simulink model "TST_ExtDem_SetPoint"  (R2016b)
settings: Solver=FixedStepDiscrete  StartTime=0.0  StopTime=simTime  FixedStep=sampleTime  RelTol=1e-3
values from neighbouring files (symbols this model uses):
  testCase = 1    [initTST_ExtDem_SetPoint_001.m]    (also in initTST_ExtDem_SetPoint_002.m = 2; initTST_ExtDem_SetPoint_003.m = 3)
libraries: simulink x13, UnitTest_Lib x9
settings Model: Creator=bianxuyin  LastModifiedBy=bianxuyin
settings DebuggingCC: SignalRangeChecking=error

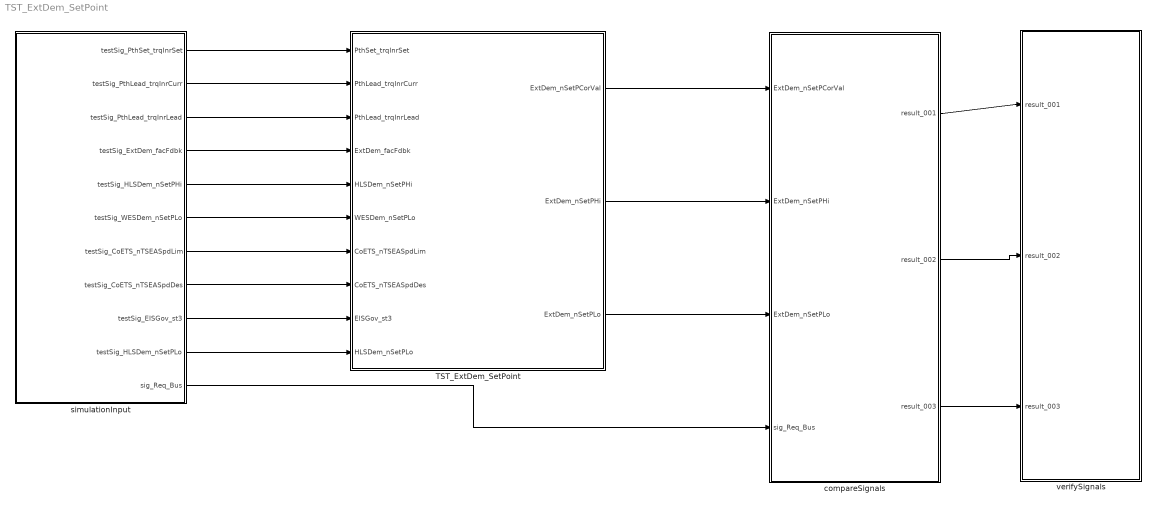
== system TST_ExtDem_SetPoint ==
  TST_ExtDem_SetPoint : Subsystem
  compareSignals : Subsystem
  simulationInput : Subsystem
  verifySignals : Subsystem
  wires:
  simulationInput/1(testSig_PthSet_trqInrSet) -> TST_ExtDem_SetPoint/1(PthSet_trqInrSet)
  simulationInput/2(testSig_PthLead_trqInrCurr) -> TST_ExtDem_SetPoint/2(PthLead_trqInrCurr)
  simulationInput/3(testSig_PthLead_trqInrLead) -> TST_ExtDem_SetPoint/3(PthLead_trqInrLead)
  simulationInput/4(testSig_ExtDem_facFdbk) -> TST_ExtDem_SetPoint/4(ExtDem_facFdbk)
  simulationInput/5(testSig_HLSDem_nSetPHi) -> TST_ExtDem_SetPoint/5(HLSDem_nSetPHi)
  simulationInput/6(testSig_WESDem_nSetPLo) -> TST_ExtDem_SetPoint/6(WESDem_nSetPLo)
  simulationInput/7(testSig_CoETS_nTSEASpdLim) -> TST_ExtDem_SetPoint/7(CoETS_nTSEASpdLim)
  simulationInput/8(testSig_CoETS_nTSEASpdDes) -> TST_ExtDem_SetPoint/8(CoETS_nTSEASpdDes)
  simulationInput/9(testSig_EISGov_st3) -> TST_ExtDem_SetPoint/9(EISGov_st3)
  simulationInput/10(testSig_HLSDem_nSetPLo) -> TST_ExtDem_SetPoint/10(HLSDem_nSetPLo)
  TST_ExtDem_SetPoint/1(ExtDem_nSetPCorVal) -> compareSignals/1(ExtDem_nSetPCorVal)
  TST_ExtDem_SetPoint/2(ExtDem_nSetPHi) -> compareSignals/2(ExtDem_nSetPHi)
  TST_ExtDem_SetPoint/3(ExtDem_nSetPLo) -> compareSignals/3(ExtDem_nSetPLo)
  simulationInput/11(sig_Req_Bus) -> compareSignals/4(sig_Req_Bus)
  compareSignals/1(result_001) -> verifySignals/1(result_001)
  compareSignals/2(result_002) -> verifySignals/2(result_002)
  compareSignals/3(result_003) -> verifySignals/3(result_003)

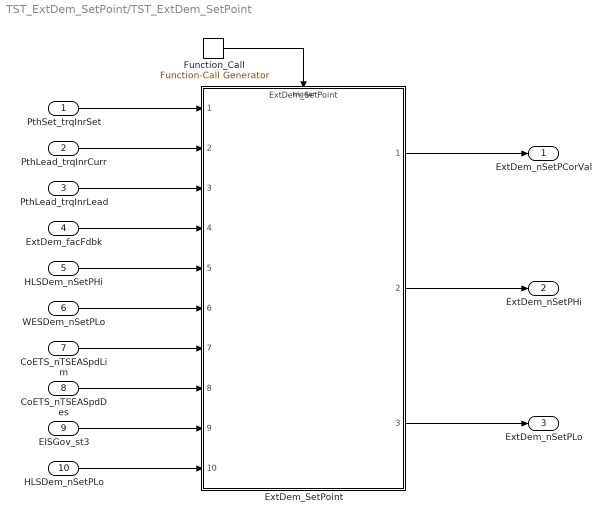
== system TST_ExtDem_SetPoint/TST_ExtDem_SetPoint ==
  PthSet_trqInrSet : Inport
  PthLead_trqInrCurr : Inport  Port=2
  PthLead_trqInrLead : Inport  Port=3
  ExtDem_facFdbk : Inport  Port=4
  HLSDem_nSetPHi : Inport  Port=5
  WESDem_nSetPLo : Inport  Port=6
  CoETS_nTSEASpdLim : Inport  Port=7
  CoETS_nTSEASpdDes : Inport  Port=8
  EISGov_st3 : Inport  Port=9
  HLSDem_nSetPLo : Inport  Port=10
  ExtDem_SetPoint : ModelReference  ModelNameDialog=ExtDem_SetPoint  SimulationMode=Normal  ModelReferenceVersion=1.39  TriggerPortName=function  TriggerPortTriggerType=function-call  TriggerPortStatesWhenEnabling=held
  Function_Call : simulink/Ports & Subsystems/Function-Call Generator  sample_time=sampleTime  numberOfIterations=1
  ExtDem_nSetPCorVal : Outport
  ExtDem_nSetPHi : Outport  Port=2
  ExtDem_nSetPLo : Outport  Port=3
  wires:
  Function_Call/1 -> ExtDem_SetPoint/Trigger
  PthSet_trqInrSet/1 -> ExtDem_SetPoint/1
  PthLead_trqInrCurr/1 -> ExtDem_SetPoint/2
  PthLead_trqInrLead/1 -> ExtDem_SetPoint/3
  ExtDem_facFdbk/1 -> ExtDem_SetPoint/4
  HLSDem_nSetPHi/1 -> ExtDem_SetPoint/5
  WESDem_nSetPLo/1 -> ExtDem_SetPoint/6
  CoETS_nTSEASpdLim/1 -> ExtDem_SetPoint/7
  CoETS_nTSEASpdDes/1 -> ExtDem_SetPoint/8
  EISGov_st3/1 -> ExtDem_SetPoint/9
  HLSDem_nSetPLo/1 -> ExtDem_SetPoint/10
  ExtDem_SetPoint/1 -> ExtDem_nSetPCorVal/1
  ExtDem_SetPoint/2 -> ExtDem_nSetPHi/1
  ExtDem_SetPoint/3 -> ExtDem_nSetPLo/1

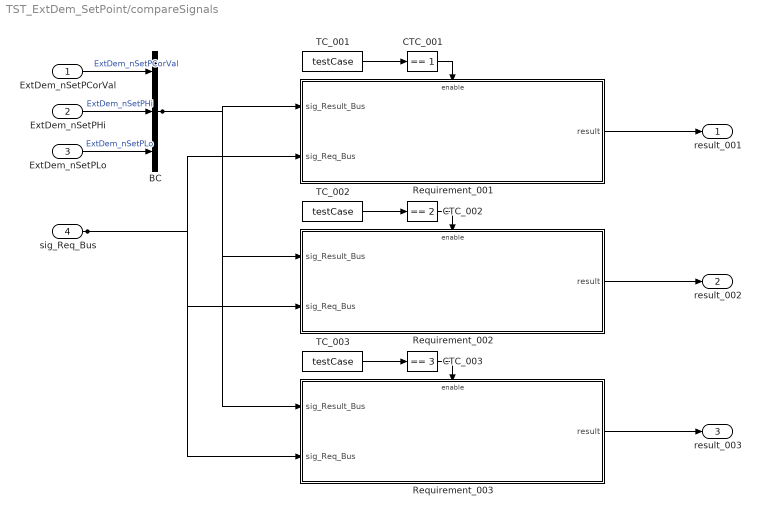
== system TST_ExtDem_SetPoint/compareSignals ==
  ExtDem_nSetPCorVal : Inport
  ExtDem_nSetPHi : Inport  Port=2
  ExtDem_nSetPLo : Inport  Port=3
  sig_Req_Bus : Inport  Port=4
  BC : BusCreator  Inputs=3
  CTC_001 : simulink/Logic and Bit Operations/Compare To Constant  relop===  const=1  OutDataTypeStr=boolean
  CTC_002 : simulink/Logic and Bit Operations/Compare To Constant  relop===  const=2  OutDataTypeStr=boolean
  CTC_003 : simulink/Logic and Bit Operations/Compare To Constant  relop===  const=3  OutDataTypeStr=boolean
  Requirement_001 : Subsystem
  Requirement_002 : Subsystem
  Requirement_003 : Subsystem
  TC_001 : Constant  Value=testCase
  TC_002 : Constant  Value=testCase
  TC_003 : Constant  Value=testCase
  result_001 : Outport
  result_002 : Outport  Port=2
  result_003 : Outport  Port=3
  wires:
  ExtDem_nSetPCorVal/1 -> BC/1  "ExtDem_nSetPCorVal"
  ExtDem_nSetPHi/1 -> BC/2  "ExtDem_nSetPHi"
  ExtDem_nSetPLo/1 -> BC/3  "ExtDem_nSetPLo"
  TC_001/1 -> CTC_001/1
  CTC_001/1 -> Requirement_001/Enable
  sig_Req_Bus/1 -> Requirement_001/2(sig_Req_Bus), Requirement_002/2(sig_Req_Bus), Requirement_003/2(sig_Req_Bus)
  BC/1 -> Requirement_001/1(sig_Result_Bus), Requirement_002/1(sig_Result_Bus), Requirement_003/1(sig_Result_Bus)
  Requirement_001/1(result) -> result_001/1
  TC_002/1 -> CTC_002/1
  CTC_002/1 -> Requirement_002/Enable
  Requirement_002/1(result) -> result_002/1
  TC_003/1 -> CTC_003/1
  CTC_003/1 -> Requirement_003/Enable
  Requirement_003/1(result) -> result_003/1

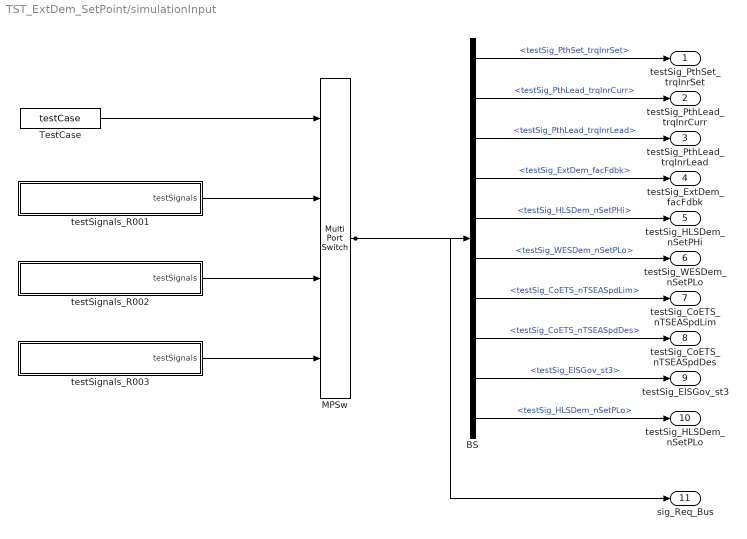
== system TST_ExtDem_SetPoint/simulationInput ==
  BS : BusSelector  OutputSignals=testSig_PthSet_trqInrSet,testSig_PthLead_trqInrCurr,testSig_PthLead_trqInrLead,testSig_ExtDem_facFdbk,testSig_HLSDem_nSetPHi,testSig_WESDem_nSetPLo,testSig_CoETS_nTSEASpdLim,testSig_CoETS_nTSEASpdDes,testSig_EISGov_st3,testSig_HLSDem_nSetPLo
  MPSw : MultiPortSwitch  SaturateOnIntegerOverflow=on  InputSameDT=on
  TestCase : Constant  Value=testCase
  testSignals_R001 : Subsystem
  testSignals_R002 : Subsystem
  testSignals_R003 : Subsystem
  testSig_PthSet_trqInrSet : Outport
  testSig_PthLead_trqInrCurr : Outport  Port=2
  testSig_PthLead_trqInrLead : Outport  Port=3
  testSig_ExtDem_facFdbk : Outport  Port=4
  testSig_HLSDem_nSetPHi : Outport  Port=5
  testSig_WESDem_nSetPLo : Outport  Port=6
  testSig_CoETS_nTSEASpdLim : Outport  Port=7
  testSig_CoETS_nTSEASpdDes : Outport  Port=8
  testSig_EISGov_st3 : Outport  Port=9
  testSig_HLSDem_nSetPLo : Outport  Port=10
  sig_Req_Bus : Outport  Port=11
  wires:
  BS/1 -> testSig_PthSet_trqInrSet/1  "<testSig_PthSet_trqInrSet>"
  BS/2 -> testSig_PthLead_trqInrCurr/1  "<testSig_PthLead_trqInrCurr>"
  BS/3 -> testSig_PthLead_trqInrLead/1  "<testSig_PthLead_trqInrLead>"
  BS/4 -> testSig_ExtDem_facFdbk/1  "<testSig_ExtDem_facFdbk>"
  BS/5 -> testSig_HLSDem_nSetPHi/1  "<testSig_HLSDem_nSetPHi>"
  BS/6 -> testSig_WESDem_nSetPLo/1  "<testSig_WESDem_nSetPLo>"
  BS/7 -> testSig_CoETS_nTSEASpdLim/1  "<testSig_CoETS_nTSEASpdLim>"
  BS/8 -> testSig_CoETS_nTSEASpdDes/1  "<testSig_CoETS_nTSEASpdDes>"
  BS/9 -> testSig_EISGov_st3/1  "<testSig_EISGov_st3>"
  BS/10 -> testSig_HLSDem_nSetPLo/1  "<testSig_HLSDem_nSetPLo>"
  MPSw/1 -> BS/1, sig_Req_Bus/1
  TestCase/1 -> MPSw/1
  testSignals_R001/1(testSignals) -> MPSw/2
  testSignals_R002/1(testSignals) -> MPSw/3
  testSignals_R003/1(testSignals) -> MPSw/4

== system TST_ExtDem_SetPoint/verifySignals ==
  result_001 : Inport
  result_002 : Inport  Port=2
  result_003 : Inport  Port=3
  Assertion_001 : Assertion  Enabled=off
  Assertion_002 : Assertion  Enabled=off
  Assertion_003 : Assertion  Enabled=off
  wires:
  result_001/1 -> Assertion_001/1
  result_002/1 -> Assertion_002/1
  result_003/1 -> Assertion_003/1

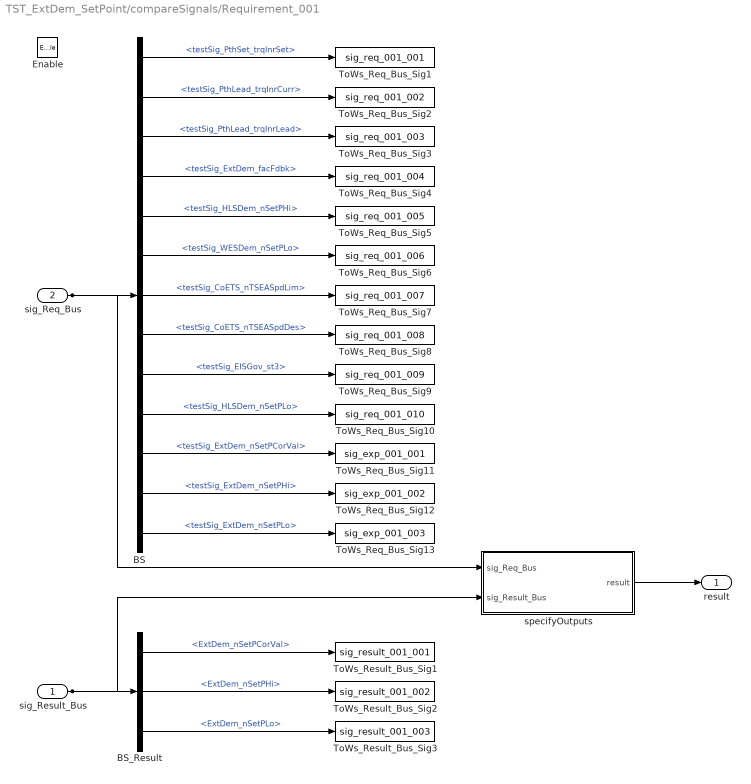
== system TST_ExtDem_SetPoint/compareSignals/Requirement_001 ==
  sig_Result_Bus : Inport
  sig_Req_Bus : Inport  Port=2
  Enable : EnablePort
  BS : BusSelector  OutputSignals=testSig_PthSet_trqInrSet,testSig_PthLead_trqInrCurr,testSig_PthLead_trqInrLead,testSig_ExtDem_facFdbk,testSig_HLSDem_nSetPHi,testSig_WESDem_nSetPLo,testSig_CoETS_nTSEASpdLim,testSig_CoETS_nTSEASpdDes,testSig_EISGov_st3,testSig_HLSDem_nSetPLo,testSig_ExtDem_nSetPCorVal,testSig_ExtDem_nSetPHi,testSig_ExtDem_nSetPLo
  BS_Result : BusSelector  OutputSignals=ExtDem_nSetPCorVal,ExtDem_nSetPHi,ExtDem_nSetPLo
  ToWs_Req_Bus_Sig1 : ToWorkspace  VariableName=sig_req_001_001  SaveFormat=Structure With Time
  ToWs_Req_Bus_Sig10 : ToWorkspace  VariableName=sig_req_001_010  SaveFormat=Structure With Time
  ToWs_Req_Bus_Sig11 : ToWorkspace  VariableName=sig_exp_001_001  SaveFormat=Structure With Time
  ToWs_Req_Bus_Sig12 : ToWorkspace  VariableName=sig_exp_001_002  SaveFormat=Structure With Time
  ToWs_Req_Bus_Sig13 : ToWorkspace  VariableName=sig_exp_001_003  SaveFormat=Structure With Time
  ToWs_Req_Bus_Sig2 : ToWorkspace  VariableName=sig_req_001_002  SaveFormat=Structure With Time
  ToWs_Req_Bus_Sig3 : ToWorkspace  VariableName=sig_req_001_003  SaveFormat=Structure With Time
  ToWs_Req_Bus_Sig4 : ToWorkspace  VariableName=sig_req_001_004  SaveFormat=Structure With Time
  ToWs_Req_Bus_Sig5 : ToWorkspace  VariableName=sig_req_001_005  SaveFormat=Structure With Time
  ToWs_Req_Bus_Sig6 : ToWorkspace  VariableName=sig_req_001_006  SaveFormat=Structure With Time
  ToWs_Req_Bus_Sig7 : ToWorkspace  VariableName=sig_req_001_007  SaveFormat=Structure With Time
  ToWs_Req_Bus_Sig8 : ToWorkspace  VariableName=sig_req_001_008  SaveFormat=Structure With Time
  ToWs_Req_Bus_Sig9 : ToWorkspace  VariableName=sig_req_001_009  SaveFormat=Structure With Time
  ToWs_Result_Bus_Sig1 : ToWorkspace  VariableName=sig_result_001_001  SaveFormat=Structure With Time
  ToWs_Result_Bus_Sig2 : ToWorkspace  VariableName=sig_result_001_002  SaveFormat=Structure With Time
  ToWs_Result_Bus_Sig3 : ToWorkspace  VariableName=sig_result_001_003  SaveFormat=Structure With Time
  specifyOutputs : Subsystem
  result : Outport
  wires:
  sig_Req_Bus/1 -> BS/1, specifyOutputs/1(sig_Req_Bus)
  BS/1 -> ToWs_Req_Bus_Sig1/1  "<testSig_PthSet_trqInrSet>"
  BS/2 -> ToWs_Req_Bus_Sig2/1  "<testSig_PthLead_trqInrCurr>"
  BS/3 -> ToWs_Req_Bus_Sig3/1  "<testSig_PthLead_trqInrLead>"
  BS/4 -> ToWs_Req_Bus_Sig4/1  "<testSig_ExtDem_facFdbk>"
  BS/5 -> ToWs_Req_Bus_Sig5/1  "<testSig_HLSDem_nSetPHi>"
  BS/6 -> ToWs_Req_Bus_Sig6/1  "<testSig_WESDem_nSetPLo>"
  BS/7 -> ToWs_Req_Bus_Sig7/1  "<testSig_CoETS_nTSEASpdLim>"
  BS/8 -> ToWs_Req_Bus_Sig8/1  "<testSig_CoETS_nTSEASpdDes>"
  BS/9 -> ToWs_Req_Bus_Sig9/1  "<testSig_EISGov_st3>"
  BS/10 -> ToWs_Req_Bus_Sig10/1  "<testSig_HLSDem_nSetPLo>"
  BS/11 -> ToWs_Req_Bus_Sig11/1  "<testSig_ExtDem_nSetPCorVal>"
  BS/12 -> ToWs_Req_Bus_Sig12/1  "<testSig_ExtDem_nSetPHi>"
  BS/13 -> ToWs_Req_Bus_Sig13/1  "<testSig_ExtDem_nSetPLo>"
  sig_Result_Bus/1 -> BS_Result/1, specifyOutputs/2(sig_Result_Bus)
  BS_Result/1 -> ToWs_Result_Bus_Sig1/1  "<ExtDem_nSetPCorVal>"
  BS_Result/2 -> ToWs_Result_Bus_Sig2/1  "<ExtDem_nSetPHi>"
  BS_Result/3 -> ToWs_Result_Bus_Sig3/1  "<ExtDem_nSetPLo>"
  specifyOutputs/1(result) -> result/1

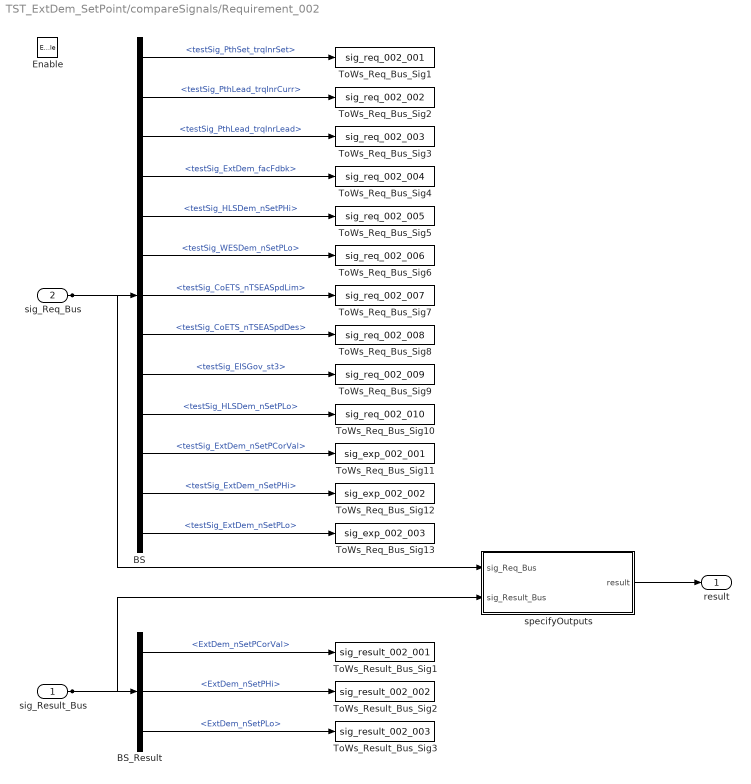
== system TST_ExtDem_SetPoint/compareSignals/Requirement_002 ==
  sig_Result_Bus : Inport
  sig_Req_Bus : Inport  Port=2
  Enable : EnablePort
  BS : BusSelector  OutputSignals=testSig_PthSet_trqInrSet,testSig_PthLead_trqInrCurr,testSig_PthLead_trqInrLead,testSig_ExtDem_facFdbk,testSig_HLSDem_nSetPHi,testSig_WESDem_nSetPLo,testSig_CoETS_nTSEASpdLim,testSig_CoETS_nTSEASpdDes,testSig_EISGov_st3,testSig_HLSDem_nSetPLo,testSig_ExtDem_nSetPCorVal,testSig_ExtDem_nSetPHi,testSig_ExtDem_nSetPLo
  BS_Result : BusSelector  OutputSignals=ExtDem_nSetPCorVal,ExtDem_nSetPHi,ExtDem_nSetPLo
  ToWs_Req_Bus_Sig1 : ToWorkspace  VariableName=sig_req_002_001  SaveFormat=Structure With Time
  ToWs_Req_Bus_Sig10 : ToWorkspace  VariableName=sig_req_002_010  SaveFormat=Structure With Time
  ToWs_Req_Bus_Sig11 : ToWorkspace  VariableName=sig_exp_002_001  SaveFormat=Structure With Time
  ToWs_Req_Bus_Sig12 : ToWorkspace  VariableName=sig_exp_002_002  SaveFormat=Structure With Time
  ToWs_Req_Bus_Sig13 : ToWorkspace  VariableName=sig_exp_002_003  SaveFormat=Structure With Time
  ToWs_Req_Bus_Sig2 : ToWorkspace  VariableName=sig_req_002_002  SaveFormat=Structure With Time
  ToWs_Req_Bus_Sig3 : ToWorkspace  VariableName=sig_req_002_003  SaveFormat=Structure With Time
  ToWs_Req_Bus_Sig4 : ToWorkspace  VariableName=sig_req_002_004  SaveFormat=Structure With Time
  ToWs_Req_Bus_Sig5 : ToWorkspace  VariableName=sig_req_002_005  SaveFormat=Structure With Time
  ToWs_Req_Bus_Sig6 : ToWorkspace  VariableName=sig_req_002_006  SaveFormat=Structure With Time
  ToWs_Req_Bus_Sig7 : ToWorkspace  VariableName=sig_req_002_007  SaveFormat=Structure With Time
  ToWs_Req_Bus_Sig8 : ToWorkspace  VariableName=sig_req_002_008  SaveFormat=Structure With Time
  ToWs_Req_Bus_Sig9 : ToWorkspace  VariableName=sig_req_002_009  SaveFormat=Structure With Time
  ToWs_Result_Bus_Sig1 : ToWorkspace  VariableName=sig_result_002_001  SaveFormat=Structure With Time
  ToWs_Result_Bus_Sig2 : ToWorkspace  VariableName=sig_result_002_002  SaveFormat=Structure With Time
  ToWs_Result_Bus_Sig3 : ToWorkspace  VariableName=sig_result_002_003  SaveFormat=Structure With Time
  specifyOutputs : Subsystem
  result : Outport
  wires:
  sig_Req_Bus/1 -> BS/1, specifyOutputs/1(sig_Req_Bus)
  BS/1 -> ToWs_Req_Bus_Sig1/1  "<testSig_PthSet_trqInrSet>"
  BS/2 -> ToWs_Req_Bus_Sig2/1  "<testSig_PthLead_trqInrCurr>"
  BS/3 -> ToWs_Req_Bus_Sig3/1  "<testSig_PthLead_trqInrLead>"
  BS/4 -> ToWs_Req_Bus_Sig4/1  "<testSig_ExtDem_facFdbk>"
  BS/5 -> ToWs_Req_Bus_Sig5/1  "<testSig_HLSDem_nSetPHi>"
  BS/6 -> ToWs_Req_Bus_Sig6/1  "<testSig_WESDem_nSetPLo>"
  BS/7 -> ToWs_Req_Bus_Sig7/1  "<testSig_CoETS_nTSEASpdLim>"
  BS/8 -> ToWs_Req_Bus_Sig8/1  "<testSig_CoETS_nTSEASpdDes>"
  BS/9 -> ToWs_Req_Bus_Sig9/1  "<testSig_EISGov_st3>"
  BS/10 -> ToWs_Req_Bus_Sig10/1  "<testSig_HLSDem_nSetPLo>"
  BS/11 -> ToWs_Req_Bus_Sig11/1  "<testSig_ExtDem_nSetPCorVal>"
  BS/12 -> ToWs_Req_Bus_Sig12/1  "<testSig_ExtDem_nSetPHi>"
  BS/13 -> ToWs_Req_Bus_Sig13/1  "<testSig_ExtDem_nSetPLo>"
  sig_Result_Bus/1 -> BS_Result/1, specifyOutputs/2(sig_Result_Bus)
  BS_Result/1 -> ToWs_Result_Bus_Sig1/1  "<ExtDem_nSetPCorVal>"
  BS_Result/2 -> ToWs_Result_Bus_Sig2/1  "<ExtDem_nSetPHi>"
  BS_Result/3 -> ToWs_Result_Bus_Sig3/1  "<ExtDem_nSetPLo>"
  specifyOutputs/1(result) -> result/1

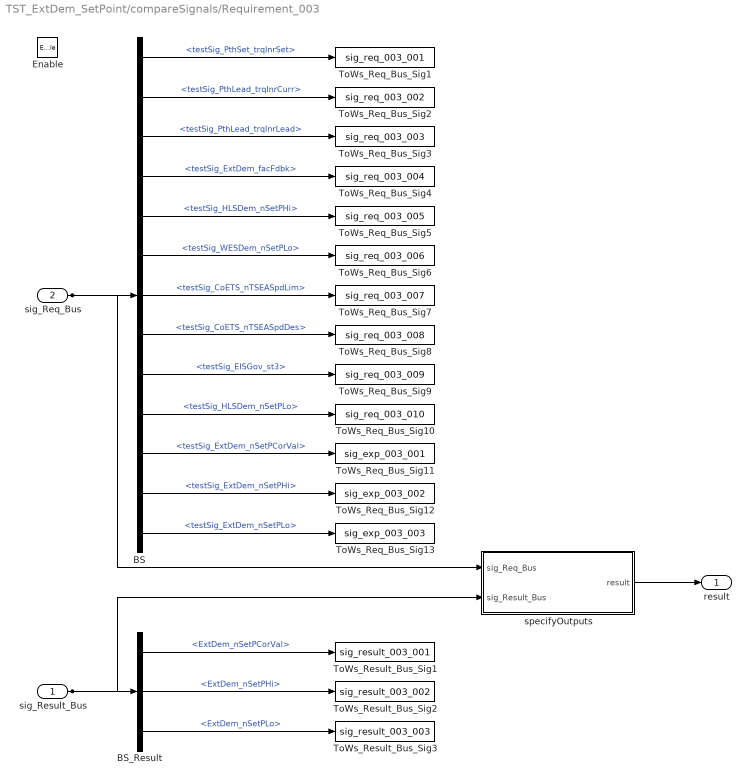
== system TST_ExtDem_SetPoint/compareSignals/Requirement_003 ==
  sig_Result_Bus : Inport
  sig_Req_Bus : Inport  Port=2
  Enable : EnablePort
  BS : BusSelector  OutputSignals=testSig_PthSet_trqInrSet,testSig_PthLead_trqInrCurr,testSig_PthLead_trqInrLead,testSig_ExtDem_facFdbk,testSig_HLSDem_nSetPHi,testSig_WESDem_nSetPLo,testSig_CoETS_nTSEASpdLim,testSig_CoETS_nTSEASpdDes,testSig_EISGov_st3,testSig_HLSDem_nSetPLo,testSig_ExtDem_nSetPCorVal,testSig_ExtDem_nSetPHi,testSig_ExtDem_nSetPLo
  BS_Result : BusSelector  OutputSignals=ExtDem_nSetPCorVal,ExtDem_nSetPHi,ExtDem_nSetPLo
  ToWs_Req_Bus_Sig1 : ToWorkspace  VariableName=sig_req_003_001  SaveFormat=Structure With Time
  ToWs_Req_Bus_Sig10 : ToWorkspace  VariableName=sig_req_003_010  SaveFormat=Structure With Time
  ToWs_Req_Bus_Sig11 : ToWorkspace  VariableName=sig_exp_003_001  SaveFormat=Structure With Time
  ToWs_Req_Bus_Sig12 : ToWorkspace  VariableName=sig_exp_003_002  SaveFormat=Structure With Time
  ToWs_Req_Bus_Sig13 : ToWorkspace  VariableName=sig_exp_003_003  SaveFormat=Structure With Time
  ToWs_Req_Bus_Sig2 : ToWorkspace  VariableName=sig_req_003_002  SaveFormat=Structure With Time
  ToWs_Req_Bus_Sig3 : ToWorkspace  VariableName=sig_req_003_003  SaveFormat=Structure With Time
  ToWs_Req_Bus_Sig4 : ToWorkspace  VariableName=sig_req_003_004  SaveFormat=Structure With Time
  ToWs_Req_Bus_Sig5 : ToWorkspace  VariableName=sig_req_003_005  SaveFormat=Structure With Time
  ToWs_Req_Bus_Sig6 : ToWorkspace  VariableName=sig_req_003_006  SaveFormat=Structure With Time
  ToWs_Req_Bus_Sig7 : ToWorkspace  VariableName=sig_req_003_007  SaveFormat=Structure With Time
  ToWs_Req_Bus_Sig8 : ToWorkspace  VariableName=sig_req_003_008  SaveFormat=Structure With Time
  ToWs_Req_Bus_Sig9 : ToWorkspace  VariableName=sig_req_003_009  SaveFormat=Structure With Time
  ToWs_Result_Bus_Sig1 : ToWorkspace  VariableName=sig_result_003_001  SaveFormat=Structure With Time
  ToWs_Result_Bus_Sig2 : ToWorkspace  VariableName=sig_result_003_002  SaveFormat=Structure With Time
  ToWs_Result_Bus_Sig3 : ToWorkspace  VariableName=sig_result_003_003  SaveFormat=Structure With Time
  specifyOutputs : Subsystem
  result : Outport
  wires:
  sig_Req_Bus/1 -> BS/1, specifyOutputs/1(sig_Req_Bus)
  BS/1 -> ToWs_Req_Bus_Sig1/1  "<testSig_PthSet_trqInrSet>"
  BS/2 -> ToWs_Req_Bus_Sig2/1  "<testSig_PthLead_trqInrCurr>"
  BS/3 -> ToWs_Req_Bus_Sig3/1  "<testSig_PthLead_trqInrLead>"
  BS/4 -> ToWs_Req_Bus_Sig4/1  "<testSig_ExtDem_facFdbk>"
  BS/5 -> ToWs_Req_Bus_Sig5/1  "<testSig_HLSDem_nSetPHi>"
  BS/6 -> ToWs_Req_Bus_Sig6/1  "<testSig_WESDem_nSetPLo>"
  BS/7 -> ToWs_Req_Bus_Sig7/1  "<testSig_CoETS_nTSEASpdLim>"
  BS/8 -> ToWs_Req_Bus_Sig8/1  "<testSig_CoETS_nTSEASpdDes>"
  BS/9 -> ToWs_Req_Bus_Sig9/1  "<testSig_EISGov_st3>"
  BS/10 -> ToWs_Req_Bus_Sig10/1  "<testSig_HLSDem_nSetPLo>"
  BS/11 -> ToWs_Req_Bus_Sig11/1  "<testSig_ExtDem_nSetPCorVal>"
  BS/12 -> ToWs_Req_Bus_Sig12/1  "<testSig_ExtDem_nSetPHi>"
  BS/13 -> ToWs_Req_Bus_Sig13/1  "<testSig_ExtDem_nSetPLo>"
  sig_Result_Bus/1 -> BS_Result/1, specifyOutputs/2(sig_Result_Bus)
  BS_Result/1 -> ToWs_Result_Bus_Sig1/1  "<ExtDem_nSetPCorVal>"
  BS_Result/2 -> ToWs_Result_Bus_Sig2/1  "<ExtDem_nSetPHi>"
  BS_Result/3 -> ToWs_Result_Bus_Sig3/1  "<ExtDem_nSetPLo>"
  specifyOutputs/1(result) -> result/1

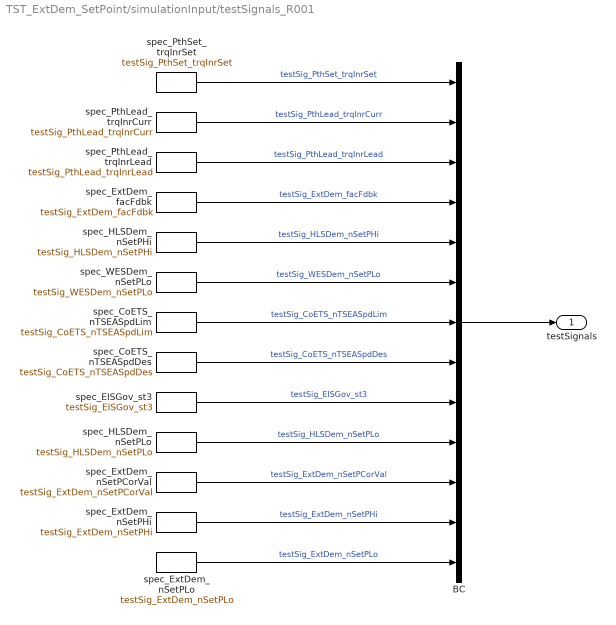
== system TST_ExtDem_SetPoint/simulationInput/testSignals_R001 ==
  BC : BusCreator  Inputs=13
  spec_CoETS_nTSEASpdDes : FromWorkspace  VariableName=testSig_CoETS_nTSEASpdDes  Interpolate=off  OutputAfterFinalValue=Holding final value
  spec_CoETS_nTSEASpdLim : FromWorkspace  VariableName=testSig_CoETS_nTSEASpdLim  Interpolate=off  OutputAfterFinalValue=Holding final value
  spec_EISGov_st3 : FromWorkspace  VariableName=testSig_EISGov_st3  Interpolate=off  OutputAfterFinalValue=Holding final value
  spec_ExtDem_facFdbk : FromWorkspace  VariableName=testSig_ExtDem_facFdbk  Interpolate=off  OutputAfterFinalValue=Holding final value
  spec_ExtDem_nSetPCorVal : FromWorkspace  VariableName=testSig_ExtDem_nSetPCorVal  Interpolate=off  OutputAfterFinalValue=Holding final value
  spec_ExtDem_nSetPHi : FromWorkspace  VariableName=testSig_ExtDem_nSetPHi  Interpolate=off  OutputAfterFinalValue=Holding final value
  spec_ExtDem_nSetPLo : FromWorkspace  VariableName=testSig_ExtDem_nSetPLo  Interpolate=off  OutputAfterFinalValue=Holding final value
  spec_HLSDem_nSetPHi : FromWorkspace  VariableName=testSig_HLSDem_nSetPHi  Interpolate=off  OutputAfterFinalValue=Holding final value
  spec_HLSDem_nSetPLo : FromWorkspace  VariableName=testSig_HLSDem_nSetPLo  Interpolate=off  OutputAfterFinalValue=Holding final value
  spec_PthLead_trqInrCurr : FromWorkspace  VariableName=testSig_PthLead_trqInrCurr  Interpolate=off  OutputAfterFinalValue=Holding final value
  spec_PthLead_trqInrLead : FromWorkspace  VariableName=testSig_PthLead_trqInrLead  Interpolate=off  OutputAfterFinalValue=Holding final value
  spec_PthSet_trqInrSet : FromWorkspace  VariableName=testSig_PthSet_trqInrSet  Interpolate=off  OutputAfterFinalValue=Holding final value
  spec_WESDem_nSetPLo : FromWorkspace  VariableName=testSig_WESDem_nSetPLo  Interpolate=off  OutputAfterFinalValue=Holding final value
  testSignals : Outport
  wires:
  BC/1 -> testSignals/1
  spec_PthSet_trqInrSet/1 -> BC/1  "testSig_PthSet_trqInrSet"
  spec_PthLead_trqInrCurr/1 -> BC/2  "testSig_PthLead_trqInrCurr"
  spec_PthLead_trqInrLead/1 -> BC/3  "testSig_PthLead_trqInrLead"
  spec_ExtDem_facFdbk/1 -> BC/4  "testSig_ExtDem_facFdbk"
  spec_HLSDem_nSetPHi/1 -> BC/5  "testSig_HLSDem_nSetPHi"
  spec_WESDem_nSetPLo/1 -> BC/6  "testSig_WESDem_nSetPLo"
  spec_CoETS_nTSEASpdLim/1 -> BC/7  "testSig_CoETS_nTSEASpdLim"
  spec_CoETS_nTSEASpdDes/1 -> BC/8  "testSig_CoETS_nTSEASpdDes"
  spec_EISGov_st3/1 -> BC/9  "testSig_EISGov_st3"
  spec_HLSDem_nSetPLo/1 -> BC/10  "testSig_HLSDem_nSetPLo"
  spec_ExtDem_nSetPCorVal/1 -> BC/11  "testSig_ExtDem_nSetPCorVal"
  spec_ExtDem_nSetPHi/1 -> BC/12  "testSig_ExtDem_nSetPHi"
  spec_ExtDem_nSetPLo/1 -> BC/13  "testSig_ExtDem_nSetPLo"

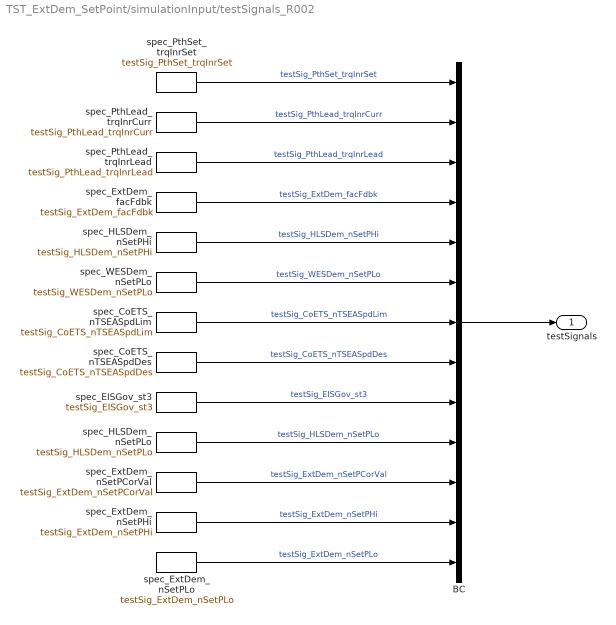
== system TST_ExtDem_SetPoint/simulationInput/testSignals_R002 ==
  BC : BusCreator  Inputs=13
  spec_CoETS_nTSEASpdDes : FromWorkspace  VariableName=testSig_CoETS_nTSEASpdDes  Interpolate=off  OutputAfterFinalValue=Holding final value
  spec_CoETS_nTSEASpdLim : FromWorkspace  VariableName=testSig_CoETS_nTSEASpdLim  Interpolate=off  OutputAfterFinalValue=Holding final value
  spec_EISGov_st3 : FromWorkspace  VariableName=testSig_EISGov_st3  Interpolate=off  OutputAfterFinalValue=Holding final value
  spec_ExtDem_facFdbk : FromWorkspace  VariableName=testSig_ExtDem_facFdbk  Interpolate=off  OutputAfterFinalValue=Holding final value
  spec_ExtDem_nSetPCorVal : FromWorkspace  VariableName=testSig_ExtDem_nSetPCorVal  Interpolate=off  OutputAfterFinalValue=Holding final value
  spec_ExtDem_nSetPHi : FromWorkspace  VariableName=testSig_ExtDem_nSetPHi  Interpolate=off  OutputAfterFinalValue=Holding final value
  spec_ExtDem_nSetPLo : FromWorkspace  VariableName=testSig_ExtDem_nSetPLo  Interpolate=off  OutputAfterFinalValue=Holding final value
  spec_HLSDem_nSetPHi : FromWorkspace  VariableName=testSig_HLSDem_nSetPHi  Interpolate=off  OutputAfterFinalValue=Holding final value
  spec_HLSDem_nSetPLo : FromWorkspace  VariableName=testSig_HLSDem_nSetPLo  Interpolate=off  OutputAfterFinalValue=Holding final value
  spec_PthLead_trqInrCurr : FromWorkspace  VariableName=testSig_PthLead_trqInrCurr  Interpolate=off  OutputAfterFinalValue=Holding final value
  spec_PthLead_trqInrLead : FromWorkspace  VariableName=testSig_PthLead_trqInrLead  Interpolate=off  OutputAfterFinalValue=Holding final value
  spec_PthSet_trqInrSet : FromWorkspace  VariableName=testSig_PthSet_trqInrSet  Interpolate=off  OutputAfterFinalValue=Holding final value
  spec_WESDem_nSetPLo : FromWorkspace  VariableName=testSig_WESDem_nSetPLo  Interpolate=off  OutputAfterFinalValue=Holding final value
  testSignals : Outport
  wires:
  BC/1 -> testSignals/1
  spec_PthSet_trqInrSet/1 -> BC/1  "testSig_PthSet_trqInrSet"
  spec_PthLead_trqInrCurr/1 -> BC/2  "testSig_PthLead_trqInrCurr"
  spec_PthLead_trqInrLead/1 -> BC/3  "testSig_PthLead_trqInrLead"
  spec_ExtDem_facFdbk/1 -> BC/4  "testSig_ExtDem_facFdbk"
  spec_HLSDem_nSetPHi/1 -> BC/5  "testSig_HLSDem_nSetPHi"
  spec_WESDem_nSetPLo/1 -> BC/6  "testSig_WESDem_nSetPLo"
  spec_CoETS_nTSEASpdLim/1 -> BC/7  "testSig_CoETS_nTSEASpdLim"
  spec_CoETS_nTSEASpdDes/1 -> BC/8  "testSig_CoETS_nTSEASpdDes"
  spec_EISGov_st3/1 -> BC/9  "testSig_EISGov_st3"
  spec_HLSDem_nSetPLo/1 -> BC/10  "testSig_HLSDem_nSetPLo"
  spec_ExtDem_nSetPCorVal/1 -> BC/11  "testSig_ExtDem_nSetPCorVal"
  spec_ExtDem_nSetPHi/1 -> BC/12  "testSig_ExtDem_nSetPHi"
  spec_ExtDem_nSetPLo/1 -> BC/13  "testSig_ExtDem_nSetPLo"

== system TST_ExtDem_SetPoint/simulationInput/testSignals_R003 ==
  BC : BusCreator  Inputs=13
  spec_CoETS_nTSEASpdDes : FromWorkspace  VariableName=testSig_CoETS_nTSEASpdDes  Interpolate=off  OutputAfterFinalValue=Holding final value
  spec_CoETS_nTSEASpdLim : FromWorkspace  VariableName=testSig_CoETS_nTSEASpdLim  Interpolate=off  OutputAfterFinalValue=Holding final value
  spec_EISGov_st3 : FromWorkspace  VariableName=testSig_EISGov_st3  Interpolate=off  OutputAfterFinalValue=Holding final value
  spec_ExtDem_facFdbk : FromWorkspace  VariableName=testSig_ExtDem_facFdbk  Interpolate=off  OutputAfterFinalValue=Holding final value
  spec_ExtDem_nSetPCorVal : FromWorkspace  VariableName=testSig_ExtDem_nSetPCorVal  Interpolate=off  OutputAfterFinalValue=Holding final value
  spec_ExtDem_nSetPHi : FromWorkspace  VariableName=testSig_ExtDem_nSetPHi  Interpolate=off  OutputAfterFinalValue=Holding final value
  spec_ExtDem_nSetPLo : FromWorkspace  VariableName=testSig_ExtDem_nSetPLo  Interpolate=off  OutputAfterFinalValue=Holding final value
  spec_HLSDem_nSetPHi : FromWorkspace  VariableName=testSig_HLSDem_nSetPHi  Interpolate=off  OutputAfterFinalValue=Holding final value
  spec_HLSDem_nSetPLo : FromWorkspace  VariableName=testSig_HLSDem_nSetPLo  Interpolate=off  OutputAfterFinalValue=Holding final value
  spec_PthLead_trqInrCurr : FromWorkspace  VariableName=testSig_PthLead_trqInrCurr  Interpolate=off  OutputAfterFinalValue=Holding final value
  spec_PthLead_trqInrLead : FromWorkspace  VariableName=testSig_PthLead_trqInrLead  Interpolate=off  OutputAfterFinalValue=Holding final value
  spec_PthSet_trqInrSet : FromWorkspace  VariableName=testSig_PthSet_trqInrSet  Interpolate=off  OutputAfterFinalValue=Holding final value
  spec_WESDem_nSetPLo : FromWorkspace  VariableName=testSig_WESDem_nSetPLo  Interpolate=off  OutputAfterFinalValue=Holding final value
  testSignals : Outport
  wires:
  BC/1 -> testSignals/1
  spec_PthSet_trqInrSet/1 -> BC/1  "testSig_PthSet_trqInrSet"
  spec_PthLead_trqInrCurr/1 -> BC/2  "testSig_PthLead_trqInrCurr"
  spec_PthLead_trqInrLead/1 -> BC/3  "testSig_PthLead_trqInrLead"
  spec_ExtDem_facFdbk/1 -> BC/4  "testSig_ExtDem_facFdbk"
  spec_HLSDem_nSetPHi/1 -> BC/5  "testSig_HLSDem_nSetPHi"
  spec_WESDem_nSetPLo/1 -> BC/6  "testSig_WESDem_nSetPLo"
  spec_CoETS_nTSEASpdLim/1 -> BC/7  "testSig_CoETS_nTSEASpdLim"
  spec_CoETS_nTSEASpdDes/1 -> BC/8  "testSig_CoETS_nTSEASpdDes"
  spec_EISGov_st3/1 -> BC/9  "testSig_EISGov_st3"
  spec_HLSDem_nSetPLo/1 -> BC/10  "testSig_HLSDem_nSetPLo"
  spec_ExtDem_nSetPCorVal/1 -> BC/11  "testSig_ExtDem_nSetPCorVal"
  spec_ExtDem_nSetPHi/1 -> BC/12  "testSig_ExtDem_nSetPHi"
  spec_ExtDem_nSetPLo/1 -> BC/13  "testSig_ExtDem_nSetPLo"

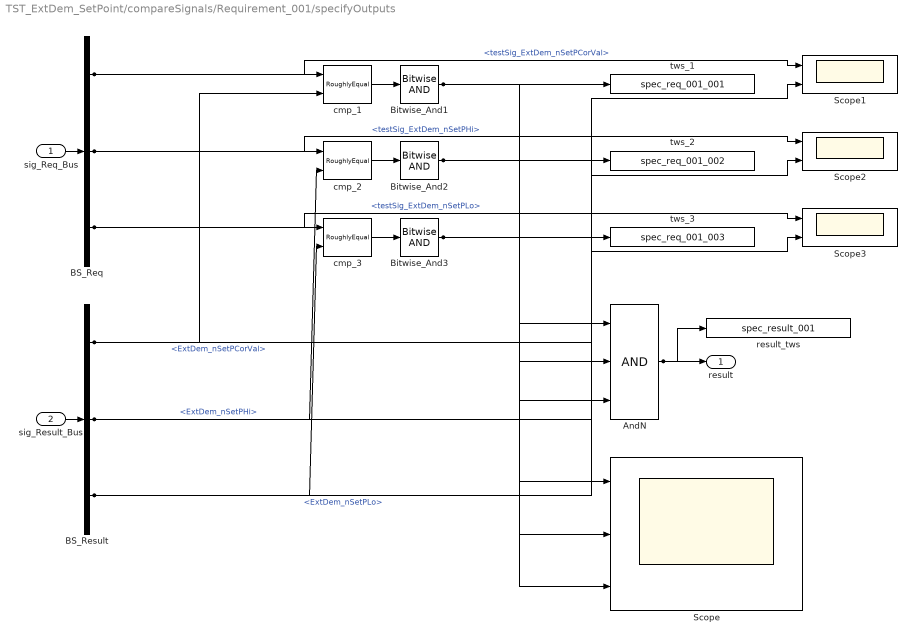
== system TST_ExtDem_SetPoint/compareSignals/Requirement_001/specifyOutputs ==
  sig_Req_Bus : Inport
  sig_Result_Bus : Inport  Port=2
  AndN : Logic  Inputs=3
  BS_Req : BusSelector  OutputSignals=testSig_ExtDem_nSetPCorVal,testSig_ExtDem_nSetPHi,testSig_ExtDem_nSetPLo
  BS_Result : BusSelector  OutputSignals=ExtDem_nSetPCorVal,ExtDem_nSetPHi,ExtDem_nSetPLo
  Bitwise_And1 : simulink/Logic and Bit Operations/Bitwise Operator  logicop=AND  UseBitMask=off  BitMask=bin2dec('11011001')  BitMaskRealWorld=Stored Integer
  Bitwise_And2 : simulink/Logic and Bit Operations/Bitwise Operator  logicop=AND  UseBitMask=off  BitMask=bin2dec('11011001')  BitMaskRealWorld=Stored Integer
  Bitwise_And3 : simulink/Logic and Bit Operations/Bitwise Operator  logicop=AND  UseBitMask=off  BitMask=bin2dec('11011001')  BitMaskRealWorld=Stored Integer
  Scope : Scope  NumInputPorts=3
  Scope1 : Scope  NumInputPorts=2
  Scope2 : Scope  NumInputPorts=2
  Scope3 : Scope  NumInputPorts=2
  cmp_1 : UnitTest_Lib/RoughlyEqual  slope=0.1
  cmp_2 : UnitTest_Lib/RoughlyEqual  slope=0.1
  cmp_3 : UnitTest_Lib/RoughlyEqual  slope=0.1
  result_tws : ToWorkspace  VariableName=spec_result_001
  tws_1 : ToWorkspace  VariableName=spec_req_001_001
  tws_2 : ToWorkspace  VariableName=spec_req_001_002
  tws_3 : ToWorkspace  VariableName=spec_req_001_003
  result : Outport
  wires:
  sig_Req_Bus/1 -> BS_Req/1
  sig_Result_Bus/1 -> BS_Result/1
  AndN/1 -> result/1, result_tws/1
  BS_Req/1 -> cmp_1/1, Scope1/1  "<testSig_ExtDem_nSetPCorVal>"
  BS_Result/1 -> cmp_1/2, Scope1/2  "<ExtDem_nSetPCorVal>"
  cmp_1/1 -> Bitwise_And1/1
  Bitwise_And1/1 -> tws_1/1, AndN/1, Scope/1
  BS_Req/2 -> cmp_2/1, Scope2/1  "<testSig_ExtDem_nSetPHi>"
  BS_Result/2 -> cmp_2/2, Scope2/2  "<ExtDem_nSetPHi>"
  cmp_2/1 -> Bitwise_And2/1
  Bitwise_And2/1 -> tws_2/1, AndN/2, Scope/2
  BS_Req/3 -> cmp_3/1, Scope3/1  "<testSig_ExtDem_nSetPLo>"
  BS_Result/3 -> cmp_3/2, Scope3/2  "<ExtDem_nSetPLo>"
  cmp_3/1 -> Bitwise_And3/1
  Bitwise_And3/1 -> tws_3/1, AndN/3, Scope/3

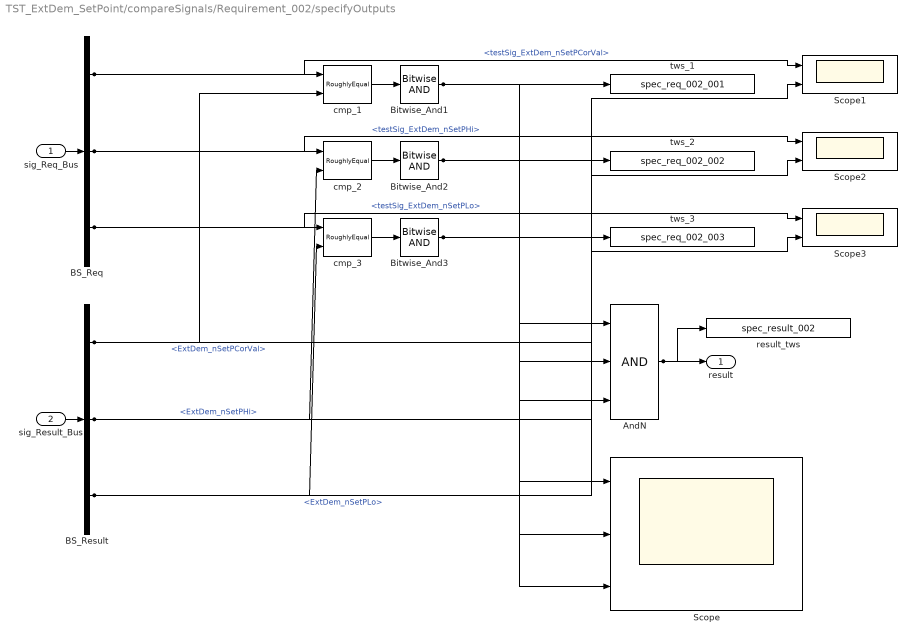
== system TST_ExtDem_SetPoint/compareSignals/Requirement_002/specifyOutputs ==
  sig_Req_Bus : Inport
  sig_Result_Bus : Inport  Port=2
  AndN : Logic  Inputs=3
  BS_Req : BusSelector  OutputSignals=testSig_ExtDem_nSetPCorVal,testSig_ExtDem_nSetPHi,testSig_ExtDem_nSetPLo
  BS_Result : BusSelector  OutputSignals=ExtDem_nSetPCorVal,ExtDem_nSetPHi,ExtDem_nSetPLo
  Bitwise_And1 : simulink/Logic and Bit Operations/Bitwise Operator  logicop=AND  UseBitMask=off  BitMask=bin2dec('11011001')  BitMaskRealWorld=Stored Integer
  Bitwise_And2 : simulink/Logic and Bit Operations/Bitwise Operator  logicop=AND  UseBitMask=off  BitMask=bin2dec('11011001')  BitMaskRealWorld=Stored Integer
  Bitwise_And3 : simulink/Logic and Bit Operations/Bitwise Operator  logicop=AND  UseBitMask=off  BitMask=bin2dec('11011001')  BitMaskRealWorld=Stored Integer
  Scope : Scope  NumInputPorts=3
  Scope1 : Scope  NumInputPorts=2
  Scope2 : Scope  NumInputPorts=2
  Scope3 : Scope  NumInputPorts=2
  cmp_1 : UnitTest_Lib/RoughlyEqual  slope=0.1
  cmp_2 : UnitTest_Lib/RoughlyEqual  slope=0.1
  cmp_3 : UnitTest_Lib/RoughlyEqual  slope=0.1
  result_tws : ToWorkspace  VariableName=spec_result_002
  tws_1 : ToWorkspace  VariableName=spec_req_002_001
  tws_2 : ToWorkspace  VariableName=spec_req_002_002
  tws_3 : ToWorkspace  VariableName=spec_req_002_003
  result : Outport
  wires:
  sig_Req_Bus/1 -> BS_Req/1
  sig_Result_Bus/1 -> BS_Result/1
  AndN/1 -> result/1, result_tws/1
  BS_Req/1 -> cmp_1/1, Scope1/1  "<testSig_ExtDem_nSetPCorVal>"
  BS_Result/1 -> cmp_1/2, Scope1/2  "<ExtDem_nSetPCorVal>"
  cmp_1/1 -> Bitwise_And1/1
  Bitwise_And1/1 -> tws_1/1, AndN/1, Scope/1
  BS_Req/2 -> cmp_2/1, Scope2/1  "<testSig_ExtDem_nSetPHi>"
  BS_Result/2 -> cmp_2/2, Scope2/2  "<ExtDem_nSetPHi>"
  cmp_2/1 -> Bitwise_And2/1
  Bitwise_And2/1 -> tws_2/1, AndN/2, Scope/2
  BS_Req/3 -> cmp_3/1, Scope3/1  "<testSig_ExtDem_nSetPLo>"
  BS_Result/3 -> cmp_3/2, Scope3/2  "<ExtDem_nSetPLo>"
  cmp_3/1 -> Bitwise_And3/1
  Bitwise_And3/1 -> tws_3/1, AndN/3, Scope/3

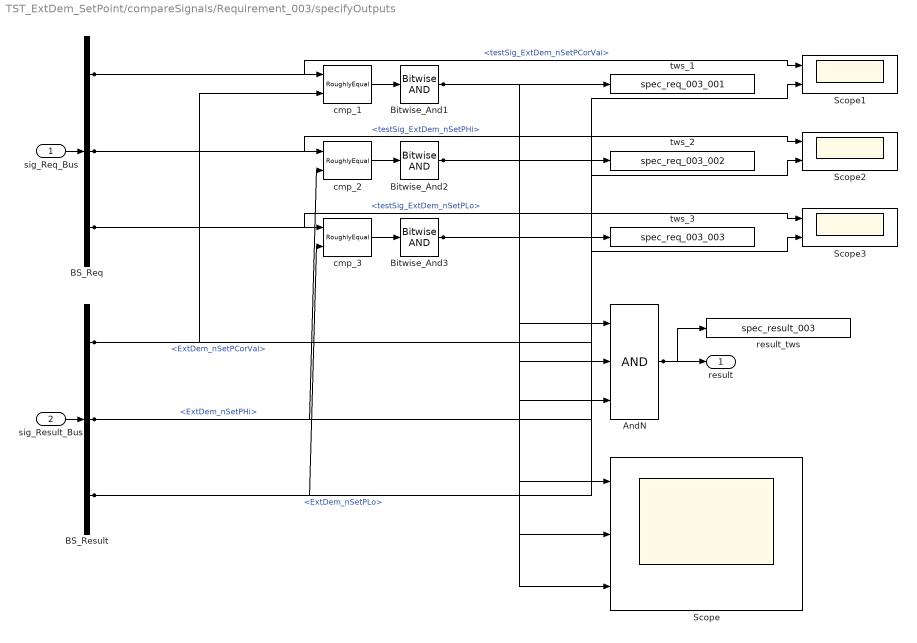
== system TST_ExtDem_SetPoint/compareSignals/Requirement_003/specifyOutputs ==
  sig_Req_Bus : Inport
  sig_Result_Bus : Inport  Port=2
  AndN : Logic  Inputs=3
  BS_Req : BusSelector  OutputSignals=testSig_ExtDem_nSetPCorVal,testSig_ExtDem_nSetPHi,testSig_ExtDem_nSetPLo
  BS_Result : BusSelector  OutputSignals=ExtDem_nSetPCorVal,ExtDem_nSetPHi,ExtDem_nSetPLo
  Bitwise_And1 : simulink/Logic and Bit Operations/Bitwise Operator  logicop=AND  UseBitMask=off  BitMask=bin2dec('11011001')  BitMaskRealWorld=Stored Integer
  Bitwise_And2 : simulink/Logic and Bit Operations/Bitwise Operator  logicop=AND  UseBitMask=off  BitMask=bin2dec('11011001')  BitMaskRealWorld=Stored Integer
  Bitwise_And3 : simulink/Logic and Bit Operations/Bitwise Operator  logicop=AND  UseBitMask=off  BitMask=bin2dec('11011001')  BitMaskRealWorld=Stored Integer
  Scope : Scope  NumInputPorts=3
  Scope1 : Scope  NumInputPorts=2
  Scope2 : Scope  NumInputPorts=2
  Scope3 : Scope  NumInputPorts=2
  cmp_1 : UnitTest_Lib/RoughlyEqual  slope=0.1
  cmp_2 : UnitTest_Lib/RoughlyEqual  slope=0.1
  cmp_3 : UnitTest_Lib/RoughlyEqual  slope=0.1
  result_tws : ToWorkspace  VariableName=spec_result_003
  tws_1 : ToWorkspace  VariableName=spec_req_003_001
  tws_2 : ToWorkspace  VariableName=spec_req_003_002
  tws_3 : ToWorkspace  VariableName=spec_req_003_003
  result : Outport
  wires:
  sig_Req_Bus/1 -> BS_Req/1
  sig_Result_Bus/1 -> BS_Result/1
  AndN/1 -> result/1, result_tws/1
  BS_Req/1 -> cmp_1/1, Scope1/1  "<testSig_ExtDem_nSetPCorVal>"
  BS_Result/1 -> cmp_1/2, Scope1/2  "<ExtDem_nSetPCorVal>"
  cmp_1/1 -> Bitwise_And1/1
  Bitwise_And1/1 -> tws_1/1, AndN/1, Scope/1
  BS_Req/2 -> cmp_2/1, Scope2/1  "<testSig_ExtDem_nSetPHi>"
  BS_Result/2 -> cmp_2/2, Scope2/2  "<ExtDem_nSetPHi>"
  cmp_2/1 -> Bitwise_And2/1
  Bitwise_And2/1 -> tws_2/1, AndN/2, Scope/2
  BS_Req/3 -> cmp_3/1, Scope3/1  "<testSig_ExtDem_nSetPLo>"
  BS_Result/3 -> cmp_3/2, Scope3/2  "<ExtDem_nSetPLo>"
  cmp_3/1 -> Bitwise_And3/1
  Bitwise_And3/1 -> tws_3/1, AndN/3, Scope/3
